simulink library "control_form_NL"  (R2023a)
settings: Solver=VariableStepAuto  StartTime=0.0  StopTime=10.0  RelTol=1e-3
undefined symbols (not defined in the file): b, d, D_rot, D_transl, eulerlimit, g, J1, J2, J3, Jr, L, m, R
settings Model: Creator=Alex  LastModifiedBy=Alex

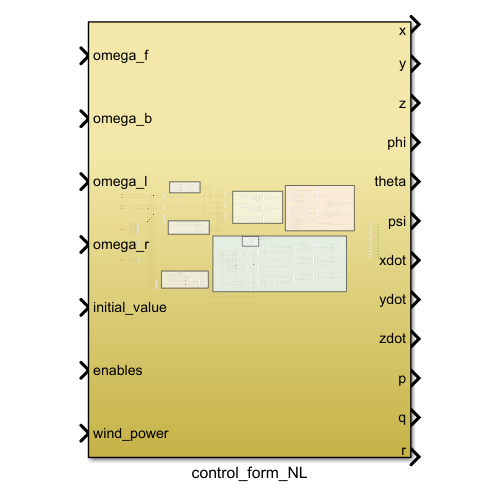
[thumbnail: Simulink's stored preview of the top-level diagram]
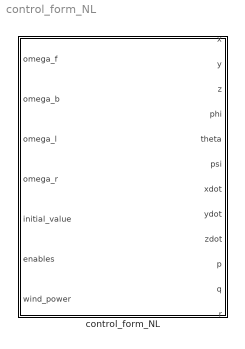
== system control_form_NL ==
  control_form_NL : Subsystem

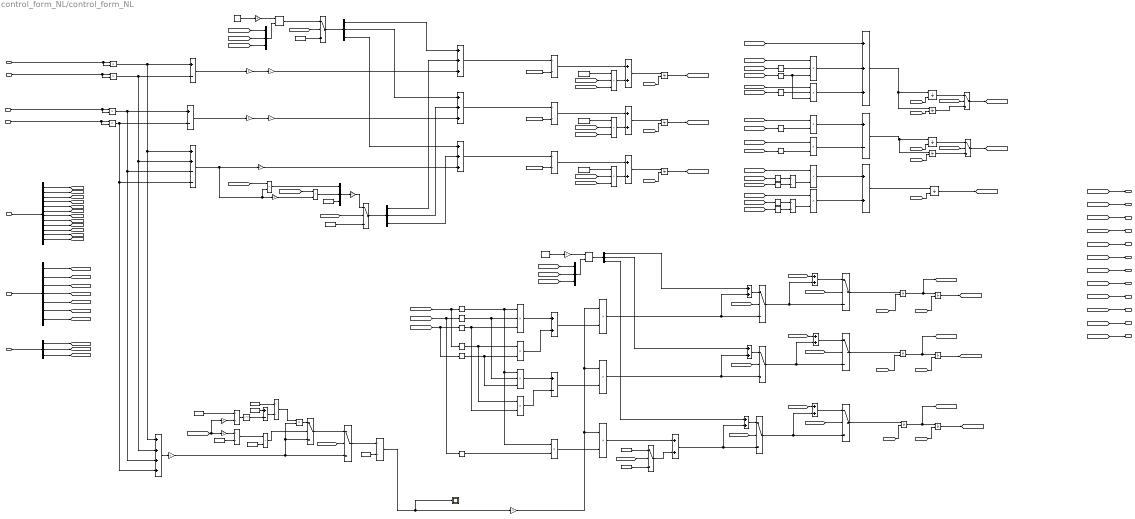
== system control_form_NL/control_form_NL ==
  note: Ground
  note: Drag torque
  note: Gyro
  note: Euler Angles
      | Rotational velocities
  note: Euler equations of motion
      | Rotational accelerations
  note: Translational dynamics
  note: Drag force
  omega_f : Inport
  omega_b : Inport  Port=2
  omega_l : Inport  Port=3
  omega_r : Inport  Port=4
  initial_value : Inport  Port=5
  enables : Inport  Port=6
  wind_power : Inport  Port=7
  Add{,1,8,19,26} (5 alike) : Sum  Inputs=+-
  Add{7,10..11,25} (4 alike) : Sum  Inputs=+++
  Add{3..5,9,18,20..24,33..34} (12 alike) : Sum
  Add2 : Sum  Inputs=++--
  Add6 : Sum  Inputs=++++
  Constant : Constant  Value=J1
  Constant1 : Constant  Value=J2
  Constant10 : Constant  Value=R
  Constant{9,11,13,20} (4 alike) : Constant  Value=0
  Constant12 : Constant  Value=D_rot
  Constant14 : Constant  Value=0.25
  Constant15 : Constant  Value=R
  Constant16 : Constant
  Constant17 : Constant
  Constant19 : Constant  Value=D_transl
  Constant2 : Constant  Value=J3
  Constant21 : Constant  Value=g
  Constant3 : Constant  Value=(J2-J3)/J1
  Constant4 : Constant  Value=(J3-J1)/J2
  Constant5 : Constant  Value=(J1-J2)/J3
  Constant6 : Constant  Value=m
  Cos : Trigonometry  Operator=cos
  Cos1 : Trigonometry  Operator=cos
  Demux : Demux  Outputs=12
  Demux1 : Demux  Outputs=7
  Demux{2..3,5..6} (4 alike) : Demux  Outputs=3
  Divide{,1..8} (9 alike) : Product  Inputs=*/
  Gain : Gain  Gain=b
  Gain1 : Gain  Gain=L
  Gain10 : Gain  Gain=4
  Gain{6,8..9,12..13} (5 alike) : Gain  Gain=-1
  Gain2 : Gain  Gain=b
  Gain3 : Gain  Gain=L
  Gain4 : Gain  Gain=d
  Gain5 : Gain  Gain=b
  Gain7 : Gain  Gain=Jr
  Integrator{,1..3,7..11,13..14} (11 alike) : Integrator  InitialConditionSource=external
  Integrator4 : Integrator  InitialConditionSource=external  LimitOutput=on  UpperSaturationLimit=eulerlimit  LowerSaturationLimit=-eulerlimit
  Integrator5 : Integrator  InitialConditionSource=external  LimitOutput=on  UpperSaturationLimit=eulerlimit  LowerSaturationLimit=-eulerlimit
  Integrator6 : Integrator  InitialConditionSource=external  LimitOutput=on  UpperSaturationLimit=pi  LowerSaturationLimit=-pi
  Mux : Mux  Inputs=3
  Mux1 : Mux  Inputs=3
  Mux3 : Mux  Inputs=3
  Product{,1..3,9..12,17..19,28,30..34} (17 alike) : Product
  Product16 : Product  Multiplication=Matrix(*)
  Product{4..8,27,29} (7 alike) : Product  Inputs=3
  Product35 : Product  Multiplication=Matrix(*)
  Relational Operator : RelationalOperator  Operator=>  OutDataTypeStr=boolean  RndMeth=Simplest  InputSameDT=off
  Scope1 : Scope
  Sin{,3..4,12,14..15} (6 alike) : Trigonometry
  Sin{1..2,5..7,13} (6 alike) : Trigonometry  Operator=cos
  Square : Math  Operator=square
  Switch{,1..5,11..17} (13 alike) : Switch  Criteria=u2 ~= 0  SaturateOnIntegerOverflow=off  InputSameDT=off
  Tan : Trigonometry  Operator=tan
  x : Outport
  y : Outport  Port=2
  z : Outport  Port=3
  phi : Outport  Port=4
  theta : Outport  Port=5
  psi : Outport  Port=6
  xdot : Outport  Port=7
  ydot : Outport  Port=8
  zdot : Outport  Port=9
  p : Outport  Port=10
  q : Outport  Port=11
  r : Outport  Port=12
  wires:
  omega_l/1 -> Product/2, Product/1
  omega_r/1 -> Product1/2, Product1/1
  Product/1 -> Add6/1, Add2/1, Add/1
  Product1/1 -> Add6/2, Add2/2, Add/2
  Add/1 -> Gain/1
  Gain/1 -> Gain1/1
  Gain1/1 -> Add25/3  "M1"
  Gain3/1 -> Add11/3  "M2"
  Gain2/1 -> Gain3/1
  Add1/1 -> Gain2/1
  Product3/1 -> Add1/2, Add6/4, Add2/4
  Product2/1 -> Add1/1, Add6/3, Add2/3
  omega_b/1 -> Product3/2, Product3/1
  omega_f/1 -> Product2/2, Product2/1
  Add2/1 -> Gain8/1, Product17/2, Gain4/1
  Gain4/1 -> Add10/3  "M3"
  Constant/1 -> Divide/2
  Constant1/1 -> Divide1/2
  Constant2/1 -> Divide2/2
  Divide/1 -> Add3/1
  Divide1/1 -> Add4/1
  Divide2/1 -> Add5/1
  Integrator/1 -> [p]  "p"
  Integrator1/1 -> [q]  "q"
  Integrator2/1 -> [r]  "r"
  Product4/1 -> Add3/2
  Product5/1 -> Add4/2
  Product6/1 -> Add5/2
  Constant3/1 -> Product4/1
  Constant4/1 -> Product5/1
  Constant5/1 -> Product6/1
  Add3/1 -> Integrator/1
  Add4/1 -> Integrator1/1
  Add5/1 -> Integrator2/1
  [q] -> Product4/2
  [r] -> Product4/3
  [r] -> Product5/2
  [p] -> Product5/3
  [p] -> Product6/2
  [q] -> Product6/3
  Add6/1 -> Gain5/1
  Gain5/1 -> Product19/2, Switch4/3, Switch2/3  "Fa"
  [p] -> Add7/1
  Product7/1 -> Add7/2
  Product8/1 -> Add7/3
  [phi] -> Sin/1
  Sin/1 -> Product7/2
  [theta] -> Tan/1
  Tan/1 -> Product8/3, Product7/3
  [phi] -> Sin1/1
  Sin1/1 -> Product8/2
  [r] -> Product8/1
  [phi] -> Sin2/1
  Sin2/1 -> Product9/2
  [q] -> Product9/1
  Product9/1 -> Add8/1
  Product10/1 -> Add8/2
  [r] -> Product10/1
  [phi] -> Sin3/1
  Sin3/1 -> Product10/2
  Divide3/1 -> Product11/2
  [q] -> Product11/1
  [r] -> Product12/1
  [phi] -> Sin4/1
  Sin4/1 -> Divide3/1
  Sin5/1 -> Divide3/2
  [theta] -> Sin5/1
  Product11/1 -> Add9/1
  Product12/1 -> Add9/2
  Divide4/1 -> Product12/2
  [phi] -> Sin6/1
  Sin6/1 -> Divide4/1
  Sin7/1 -> Divide4/2
  [theta] -> Sin7/1
  Constant6/1 -> Divide5/2
  [x] -> x/1
  [y] -> y/1
  [r] -> r/1
  [q] -> q/1
  [p] -> p/1
  [zdot] -> zdot/1
  [ydot] -> ydot/1
  [xdot] -> xdot/1
  [psi] -> psi/1
  [theta] -> theta/1
  [phi] -> phi/1
  [z] -> z/1
  Divide5/1 -> Scope1/1, Gain12/1
  [q] -> Product7/1
  initial_value/1 -> Demux/1
  Demux/1 -> [x0]
  Demux/2 -> [y0]
  Demux/3 -> [z0]
  Demux/4 -> [phi0]
  Demux/5 -> [theta0]
  Demux/6 -> [psi0]
  Demux/7 -> [xdot0]
  Demux/8 -> [ydot0]
  Demux/9 -> [zdot0]
  Demux/10 -> [p0]
  Demux/11 -> [q0]
  Demux/12 -> [r0]
  [p0] -> Integrator/2
  [q0] -> Integrator1/2
  [r0] -> Integrator2/2
  enables/1 -> Demux1/1
  Demux1/1 -> [Ena_gravity]
  Demux1/3 -> [Ena_gyro]
  Demux1/4 -> [Ena_ground]
  Demux1/5 -> [Ena_drag_force]
  Demux1/6 -> [Ena_drag_torque]
  Demux1/7 -> [Ena_wind]
  wind_power/1 -> Demux5/1
  Add10/1 -> Divide2/1  "tau3"
  Add11/1 -> Divide1/1  "tau2"
  Add25/1 -> Divide/1  "tau1"
  [Ena_gyro] -> Switch1/2
  [Ena_drag_torque] -> Switch3/2
  Constant9/1 -> Switch3/3
  Constant11/1 -> Switch1/3
  Constant12/1 -> Gain6/1
  Gain6/1 -> Product16/1
  [q] -> Mux/2
  [p] -> Mux/1
  [r] -> Mux/3
  Mux/1 -> Product16/2
  Product16/1 -> Switch3/1
  Switch3/1 -> Demux2/1  "drag_torque"
  Switch1/1 -> Demux3/1  "gyro"
  [q] -> Product17/1
  [p] -> Product18/1
  Product17/1 -> Mux1/1
  Product18/1 -> Mux1/2
  Constant13/1 -> Mux1/3
  Mux1/1 -> Gain7/1
  Gain7/1 -> Switch1/1
  Gain8/1 -> Product18/2
  Demux3/3 -> Add10/2
  Demux3/2 -> Add11/2
  Demux3/1 -> Add25/2
  Demux2/2 -> Add11/1
  [Ena_ground] -> Switch2/2
  Switch2/1 -> Divide5/1  "ground"
  Switch4/1 -> Switch2/1
  [z] -> Gain10/1, Gain9/1
  Gain9/1 -> Divide6/1
  Divide6/1 -> Relational Operator/1
  Constant10/1 -> Divide6/2
  Relational Operator/1 -> Switch4/2
  Constant14/1 -> Relational Operator/2
  Product19/1 -> Switch4/1
  Constant15/1 -> Divide7/1
  Gain10/1 -> Divide7/2
  Divide7/1 -> Square/1
  Square/1 -> Add26/2
  Constant16/1 -> Add26/1
  Divide8/1 -> Product19/1
  Add26/1 -> Divide8/2
  Constant17/1 -> Divide8/1
  Demux2/1 -> Add25/1
  Demux2/3 -> Add10/1
  Demux5/1 -> [wind_x]
  Demux5/2 -> [wind_y]
  Demux5/3 -> [wind_z]
  Switch12/1 -> Integrator3/1
  Product30/1 -> Add19/2
  [z0] -> Integrator11/2
  Sin15/1 -> Product28/1, Product30/1
  Sin12/1 -> Product28/2, Product29/3
  Integrator9/1 -> [ydot], Integrator13/1
  Switch17/1 -> Integrator9/1
  Switch16/1 -> Integrator10/1
  [phi] -> Cos/1, Sin15/1
  Sin14/1 -> Product27/2, Product29/2
  Cos/1 -> Product27/1, Product29/1, Product31/1
  Product29/1 -> Add19/1
  [ydot0] -> Integrator9/2
  Integrator14/1 -> [x]
  [y0] -> Integrator13/2
  Sin13/1 -> Product31/2
  Integrator3/1 -> [xdot], Integrator14/1
  Add19/1 -> Product33/2
  Product28/1 -> Add18/2
  [xdot0] -> Integrator3/2
  [zdot0] -> Integrator10/2
  Product34/1 -> Add20/1
  Integrator10/1 -> [zdot], Integrator11/1
  Integrator11/1 -> [z]
  Product31/1 -> Product34/2
  [psi] -> Sin12/1, Cos1/1
  Add18/1 -> Product32/2
  [theta] -> Sin14/1, Sin13/1
  Integrator13/1 -> [y]
  [x0] -> Integrator14/2
  Product27/1 -> Add18/1
  Cos1/1 -> Product27/3, Product30/2
  Gain12/1 -> Product32/1, Product33/1, Product34/1
  Constant20/1 -> Switch11/3
  Constant21/1 -> Switch11/1
  [Ena_gravity] -> Switch11/2
  Switch11/1 -> Add20/2  "gravity"
  Demux6/1 -> Add23/1
  [wind_z] -> Add34/1
  [wind_y] -> Add33/1
  [wind_x] -> Add24/1
  Add34/1 -> Switch16/1
  Add33/1 -> Switch17/1
  Add24/1 -> Switch12/1
  [Ena_wind] -> Switch12/2
  [Ena_wind] -> Switch16/2
  [Ena_wind] -> Switch17/2
  Switch15/1 -> Switch12/3, Add24/2
  Switch14/1 -> Switch17/3, Add33/2
  Switch13/1 -> Switch16/3, Add34/2
  Demux6/3 -> Add21/1
  Demux6/2 -> Add22/1
  Product35/1 -> Demux6/1
  Add23/1 -> Switch15/1
  Product32/1 -> Add23/2, Switch15/3
  [Ena_drag_force] -> Switch15/2
  [Ena_drag_force] -> Switch14/2
  Product33/1 -> Add22/2, Switch14/3
  Add22/1 -> Switch14/1
  [ydot] -> Mux3/2
  Constant19/1 -> Gain13/1
  Gain13/1 -> Product35/1
  [xdot] -> Mux3/1
  [zdot] -> Mux3/3
  Mux3/1 -> Product35/2
  Add21/1 -> Switch13/1
  Add20/1 -> Switch13/3, Add21/2
  [Ena_drag_force] -> Switch13/2
  Demux1/2 -> [Ena_euler_sat]
  Add7/1 -> Integrator8/1, Integrator4/1  "phidot"
  Add8/1 -> Integrator7/1, Integrator5/1  "thetadot"
  [phi0] -> Integrator8/2
  [theta0] -> Integrator5/2
  Integrator4/1 -> Switch5/1  "phi_lim"
  [Ena_euler_sat] -> Switch5/2
  Add9/1 -> Integrator6/1  "psidot"
  Switch5/1 -> [phi]  "phi"
  Integrator7/1 -> Switch/3  "theta_nolim"
  Integrator6/1 -> [psi]  "psi"
  [theta0] -> Integrator7/2
  Switch/1 -> [theta]  "theta"
  [Ena_euler_sat] -> Switch/2
  Integrator5/1 -> Switch/1  "theta_lim"
  Integrator8/1 -> Switch5/3  "phi_nolim"
  [phi0] -> Integrator4/2
  [psi0] -> Integrator6/2
